simulink model "untitled1"  (R2024a)
settings: Solver=VariableStepAuto  StartTime=0.0  StopTime=10  RelTol=1e-3
values from neighbouring files (symbols this model uses):
  A = jacobian(f, [q;w])    [dynamics.m]    (also in dynamics_ext.m = jacobian(f,[w1;g1;w2;g2;w3;g3;b1;b2]); dynamics_new.m = jacobian(f,[w;g]))
  B = jacobian(f, tau)    [dynamics.m]    (also in dynamics_ext.m = jacobian(f,[u_1;u_2]); dynamics_new.m = jacobian(f,u))
  C = eye(length(A))    [main.m]
  D = zeros(7,3)    [main.m]
  K = control_sys(A,B)    [main.m]
libraries: aerolibutil x2
settings Model: Creator=Floatsat  LastModifiedBy=Floatsat

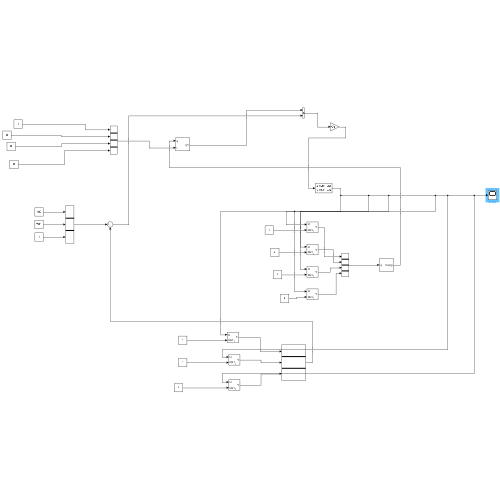
[thumbnail: Simulink's stored preview of the top-level diagram]
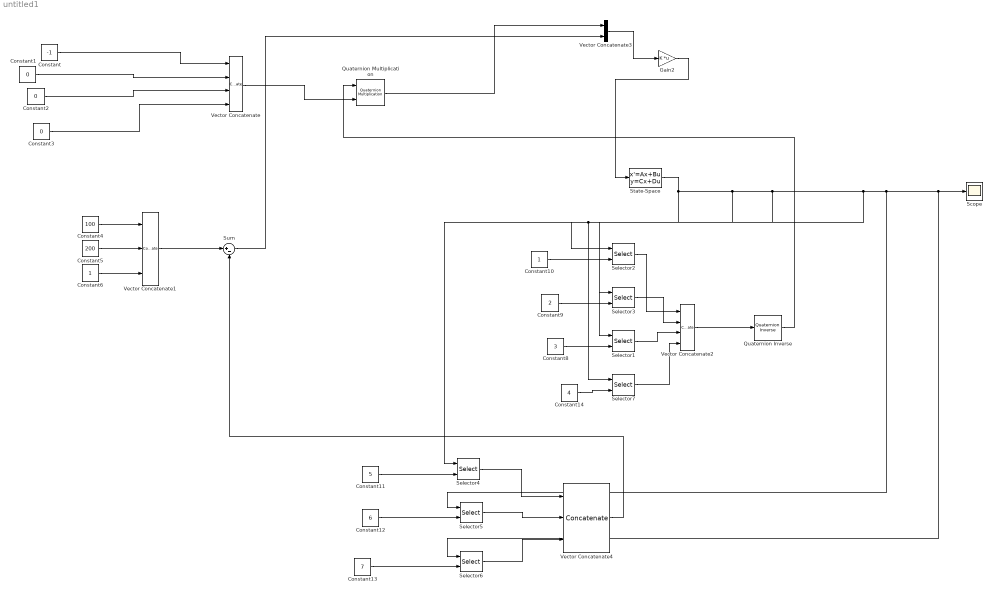
== system untitled1 ==
  Constant : Constant  Value=-1
  Constant1 : Constant  Value=0
  Constant10 : Constant
  Constant11 : Constant  Value=5
  Constant12 : Constant  Value=6
  Constant13 : Constant  Value=7
  Constant14 : Constant  Value=4
  Constant2 : Constant  Value=0
  Constant3 : Constant  Value=0
  Constant4 : Constant  Value=100
  Constant5 : Constant  Value=200
  Constant6 : Constant
  Constant8 : Constant  Value=3
  Constant9 : Constant  Value=2
  Gain2 : Gain  Gain=K  Multiplication=Matrix(K*u)
  Quaternion Inverse : aerolibutil/Quaternion Inverse
  Quaternion Multiplication : aerolibutil/Quaternion Multiplication
  Scope : Scope
  Selector{1..7} (7 alike) : Selector  InputPortWidth=7  IndexOptions=Index vector (port)  Indices=[1 3]  OutputSizes=1
  State-Space : StateSpace  A=A  B=B  C=C  D=D  InitialCondition=[-1; 0; 0; 0; 100; 0;0]
  Sum : Sum  Inputs=|+-
  Vector Concatenate : Concatenate  NumInputs=4
  Vector Concatenate1 : Concatenate  NumInputs=3
  Vector Concatenate2 : Concatenate  NumInputs=4
  Vector Concatenate3 : Concatenate
  Vector Concatenate4 : Concatenate  NumInputs=3
  wires:
  Vector Concatenate1/1 -> Sum/1
  Selector6/1 -> Vector Concatenate4/3
  State-Space/1 -> Selector2/1, Selector3/1, Selector1/1, Selector4/1, Selector7/1, Selector5/1, Scope/1, Selector6/1
  Selector1/1 -> Vector Concatenate2/3
  Constant12/1 -> Selector5/2
  Selector2/1 -> Vector Concatenate2/1
  Constant10/1 -> Selector2/2
  Selector5/1 -> Vector Concatenate4/2
  Constant8/1 -> Selector1/2
  Constant11/1 -> Selector4/2
  Constant4/1 -> Vector Concatenate1/1
  Constant2/1 -> Vector Concatenate/3
  Constant1/1 -> Vector Concatenate/2
  Constant9/1 -> Selector3/2
  Constant5/1 -> Vector Concatenate1/2
  Gain2/1 -> State-Space/1
  Constant/1 -> Vector Concatenate/1
  Vector Concatenate4/1 -> Sum/2
  Vector Concatenate3/1 -> Gain2/1
  Constant13/1 -> Selector6/2
  Constant6/1 -> Vector Concatenate1/3
  Selector3/1 -> Vector Concatenate2/2
  Selector4/1 -> Vector Concatenate4/1
  Sum/1 -> Vector Concatenate3/2
  Constant3/1 -> Vector Concatenate/4
  Constant14/1 -> Selector7/2
  Selector7/1 -> Vector Concatenate2/4
  Vector Concatenate2/1 -> Quaternion Inverse/1
  Quaternion Inverse/1 -> Quaternion Multiplication/1
  Vector Concatenate/1 -> Quaternion Multiplication/2
  Quaternion Multiplication/1 -> Vector Concatenate3/1
